simulink model "PID_control_Model_square_input"  (R2022a)
settings: Solver=VariableStepAuto  StartTime=0.0  StopTime=100  RelTol=1e-3
values from neighbouring files (symbols this model uses):
  b1_damp = 0.5    [variable_for_simulink.m]
  b2_damp = 0.5    [variable_for_simulink.m]
  center1 = 0.216    [variable_for_simulink.m]
  center2 = 0.216    [variable_for_simulink.m]
  gravity = 9.8    [variable_for_simulink.m]
  inertia1 = 0.247    [variable_for_simulink.m]
  inertia2 = 0.177    [variable_for_simulink.m]
  length1 = 0.432    [variable_for_simulink.m]
  mass1 = 15.91    [variable_for_simulink.m]
  mass2 = 11.36    [variable_for_simulink.m]
libraries: slpidlib x2
settings Model: Creator=Steve  LastModifiedBy=Steve

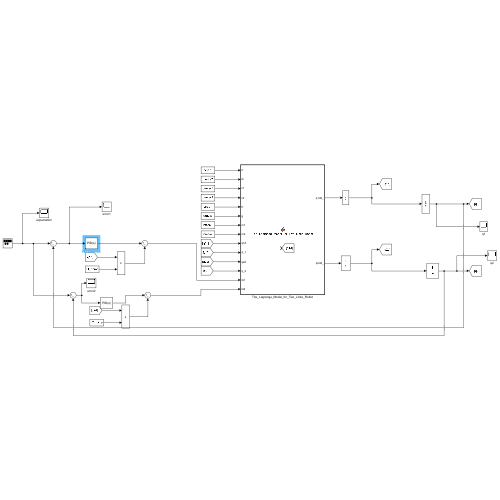
[thumbnail: Simulink's stored preview of the top-level diagram]
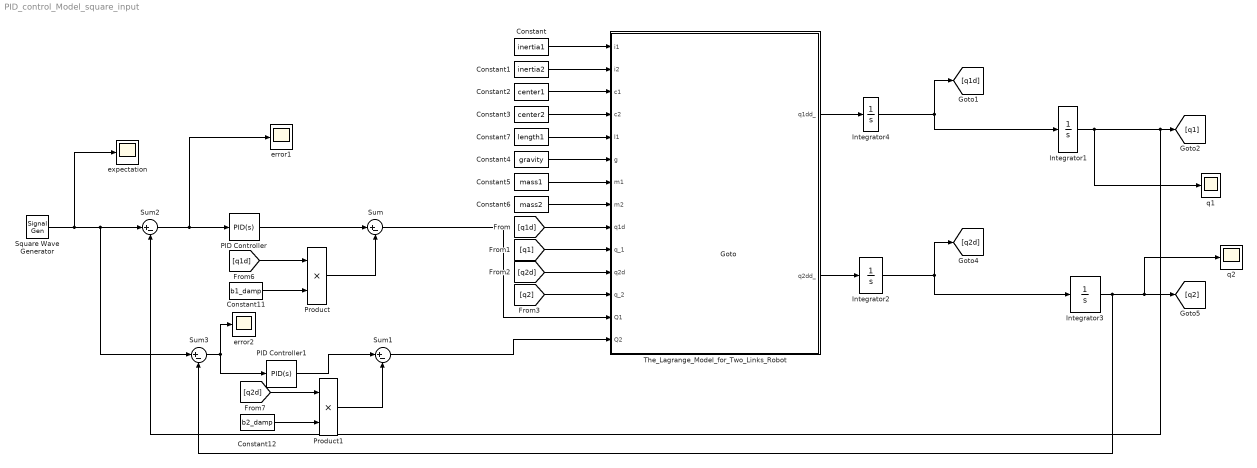
== system PID_control_Model_square_input ==
  Constant : Constant  Value=inertia1
  Constant1 : Constant  Value=inertia2
  Constant11 : Constant  Value=b1_damp
  Constant12 : Constant  Value=b2_damp
  Constant2 : Constant  Value=center1
  Constant3 : Constant  Value=center2
  Constant4 : Constant  Value=gravity
  Constant5 : Constant  Value=mass1
  Constant6 : Constant  Value=mass2
  Constant7 : Constant  Value=length1
  Integrator1 : Integrator  InitialCondition=1
  Integrator2 : Integrator
  Integrator3 : Integrator  InitialCondition=1
  Integrator4 : Integrator
  PID Controller : slpidlib/PID Controller  Controller=PID  Form=Parallel  TimeDomain=Continuous-time  UseExternalTs=off  SampleTime=-1  IntegratorMethod=Forward Euler  FilterMethod=Forward Euler  ControllerParametersSource=internal  P=100  I=50  UseKiTs=off  D=1  N=100  UseFilter=on  TunerSelectOption=Frequency Response Based  InitialConditionSource=internal  InitialConditionForIntegrator=0  InitialConditionForFilter=0  DifferentiatorICPrevScaledInput=0  ExternalReset=none  TrackingMode=off  Kt=1  LimitOutput=off  SatLimitsSource=internal  UpperSaturationLimit=inf  LowerSaturationLimit=-inf  LinearizeAsGain=on  AntiWindupMode=none  Kb=1  POutMin=[]  POutMax=[]  IOutMin=[]  IOutMax=[]  DOutMin=[]  DOutMax=[]  NOutMin=[]  NOutMax=[]  SumOutMin=[]  SumOutMax=[]  SaturationOutMin=[]  SaturationOutMax=[]  PParamMin=[]  PParamMax=[]  IParamMin=[]  IParamMax=[]  DParamMin=[]  DParamMax=[]  NParamMin=[]  NParamMax=[]  KbParamMin=[]  KbParamMax=[]  KtParamMin=[]  KtParamMax=[]  KbOutMin=[]  KbOutMax=[]  KtOutMin=[]  KtOutMax=[]  IntegratorOutMin=[]  IntegratorOutMax=[]  FilterOutMin=[]  FilterOutMax=[]  SumI1OutMin=[]  SumI1OutMax=[]  SumI2OutMin=[]  SumI2OutMax=[]  SumI3OutMin=[]  SumI3OutMax=[]  SumI4OutMin=[]  SumI4OutMax=[]  SumDOutMin=[]  SumDOutMax=[]  DifferentiatorOutMin=[]  DifferentiatorOutMax=[]  FilterDiffOutCoefMin=[]  FilterDiffOutCoefMax=[]  ReciprocalOutMin=[]  ReciprocalOutMax=[]  SumDenOutMin=[]  SumDenOutMax=[]  SumNumOutMin=[]  SumNumOutMax=[]  DivideOutMin=[]  DivideOutMax=[]  UdiffTsProdOutMin=[]  UdiffTsProdOutMax=[]  NTsProdOutMin=[]  NTsProdOutMax=[]  UintegralTsProdOutMin=[]  UintegralTsProdOutMax=[]  UngainTsProdOutMin=[]  UngainTsProdOutMax=[]  IntegratorContinuousStateAttributes=''  IntegratorStateMustResolveToSignalObject=off  IntegratorRTWStateStorageClass=Auto  FilterContinuousStateAttributes=''  FilterStateMustResolveToSignalObject=off  FilterRTWStateStorageClass=Auto  ParallelPVariant=InternalParameters  IdealPVariant=Disabled  IVariant=InternalParameters  DVariant=InternalParameters  IntegratorVariant=Continuous  SatVariant=Disabled  AWVariant=Passthrough  PCopyVariant=Disabled  TRVariant=Disabled  FdbkBlocksVariant=Forward  IdealPFdbkVariant=Disabled  SatFdbkVariant=Disabled  DerivativeFilterVariant=ContFilter  NVariant=InternalParameters  NCopyVariant=Disabled  FilterICVariant=InternalICsFilter  IntegratorICVariant=InternalICs  ExternalResetVariant=Disabled  TRSumVariant=Passthrough  SumFdbkVariant=Disabled  SumVariant=Sum_PID  TsampFilterVariant=InternalTs  TsampNgainVariant=Passthrough  TsampIntegralVariant=Passthrough  ExternalSaturationOutDataTypeStr=Inherit: Same as second input  aMode=0
  PID Controller1 : slpidlib/PID Controller  Controller=PID  Form=Parallel  TimeDomain=Continuous-time  UseExternalTs=off  SampleTime=-1  IntegratorMethod=Forward Euler  FilterMethod=Forward Euler  ControllerParametersSource=internal  P=100  I=50  UseKiTs=off  D=20  N=100  UseFilter=on  TunerSelectOption=Transfer Function Based (PID Tuner App)  InitialConditionSource=internal  InitialConditionForIntegrator=0  InitialConditionForFilter=0  DifferentiatorICPrevScaledInput=0  ExternalReset=none  TrackingMode=off  Kt=1  LimitOutput=off  SatLimitsSource=internal  UpperSaturationLimit=inf  LowerSaturationLimit=-inf  LinearizeAsGain=on  AntiWindupMode=none  Kb=1  POutMin=[]  POutMax=[]  IOutMin=[]  IOutMax=[]  DOutMin=[]  DOutMax=[]  NOutMin=[]  NOutMax=[]  SumOutMin=[]  SumOutMax=[]  SaturationOutMin=[]  SaturationOutMax=[]  PParamMin=[]  PParamMax=[]  IParamMin=[]  IParamMax=[]  DParamMin=[]  DParamMax=[]  NParamMin=[]  NParamMax=[]  KbParamMin=[]  KbParamMax=[]  KtParamMin=[]  KtParamMax=[]  KbOutMin=[]  KbOutMax=[]  KtOutMin=[]  KtOutMax=[]  IntegratorOutMin=[]  IntegratorOutMax=[]  FilterOutMin=[]  FilterOutMax=[]  SumI1OutMin=[]  SumI1OutMax=[]  SumI2OutMin=[]  SumI2OutMax=[]  SumI3OutMin=[]  SumI3OutMax=[]  SumI4OutMin=[]  SumI4OutMax=[]  SumDOutMin=[]  SumDOutMax=[]  DifferentiatorOutMin=[]  DifferentiatorOutMax=[]  FilterDiffOutCoefMin=[]  FilterDiffOutCoefMax=[]  ReciprocalOutMin=[]  ReciprocalOutMax=[]  SumDenOutMin=[]  SumDenOutMax=[]  SumNumOutMin=[]  SumNumOutMax=[]  DivideOutMin=[]  DivideOutMax=[]  UdiffTsProdOutMin=[]  UdiffTsProdOutMax=[]  NTsProdOutMin=[]  NTsProdOutMax=[]  UintegralTsProdOutMin=[]  UintegralTsProdOutMax=[]  UngainTsProdOutMin=[]  UngainTsProdOutMax=[]  IntegratorContinuousStateAttributes=''  IntegratorStateMustResolveToSignalObject=off  IntegratorRTWStateStorageClass=Auto  FilterContinuousStateAttributes=''  FilterStateMustResolveToSignalObject=off  FilterRTWStateStorageClass=Auto  ParallelPVariant=InternalParameters  IdealPVariant=Disabled  IVariant=InternalParameters  DVariant=InternalParameters  IntegratorVariant=Continuous  SatVariant=Disabled  AWVariant=Passthrough  PCopyVariant=Disabled  TRVariant=Disabled  FdbkBlocksVariant=Forward  IdealPFdbkVariant=Disabled  SatFdbkVariant=Disabled  DerivativeFilterVariant=ContFilter  NVariant=InternalParameters  NCopyVariant=Disabled  FilterICVariant=InternalICsFilter  IntegratorICVariant=InternalICs  ExternalResetVariant=Disabled  TRSumVariant=Passthrough  SumFdbkVariant=Disabled  SumVariant=Sum_PID  TsampFilterVariant=InternalTs  TsampNgainVariant=Passthrough  TsampIntegralVariant=Passthrough  ExternalSaturationOutDataTypeStr=Inherit: Same as second input  aMode=0
  Product : Product
  Product1 : Product
  Square Wave Generator : SignalGenerator  WaveForm=square  Units=rad/sec
  Sum{,1..3} (4 alike) : Sum  Inputs=|+-
  The_Lagrange_Model_for_Two_Links_Robot : MATLAB Function  TreatAsAtomicUnit=on
  error1 : Scope
  error2 : Scope
  expectation : Scope
  q1 : Scope
  q2 : Scope
  wires:
  Constant4/1 -> The_Lagrange_Model_for_Two_Links_Robot/6(g)
  Constant1/1 -> The_Lagrange_Model_for_Two_Links_Robot/2(i2)
  Constant3/1 -> The_Lagrange_Model_for_Two_Links_Robot/4(c2)
  Constant/1 -> The_Lagrange_Model_for_Two_Links_Robot/1(i1)
  Constant2/1 -> The_Lagrange_Model_for_Two_Links_Robot/3(c1)
  Constant7/1 -> The_Lagrange_Model_for_Two_Links_Robot/5(l1)
  Constant5/1 -> The_Lagrange_Model_for_Two_Links_Robot/7(m1)
  Constant6/1 -> The_Lagrange_Model_for_Two_Links_Robot/8(m2)
  [q1d] -> The_Lagrange_Model_for_Two_Links_Robot/9(q1d)
  [q1] -> The_Lagrange_Model_for_Two_Links_Robot/10(q_1)
  [q2d] -> The_Lagrange_Model_for_Two_Links_Robot/11(q2d)
  [q2] -> The_Lagrange_Model_for_Two_Links_Robot/12(q_2)
  Integrator4/1 -> [q1d], Integrator1/1
  [q2d] -> Product1/1
  Integrator2/1 -> Integrator3/1, [q2d]
  Constant12/1 -> Product1/2
  Integrator1/1 -> Sum2/2, [q1], q1/1
  Integrator3/1 -> [q2], q2/1, Sum3/2
  Product/1 -> Sum/2
  [q1d] -> Product/1
  Constant11/1 -> Product/2
  Product1/1 -> Sum1/2
  The_Lagrange_Model_for_Two_Links_Robot/1(q1dd_) -> Integrator4/1
  The_Lagrange_Model_for_Two_Links_Robot/2(q2dd_) -> Integrator2/1
  Sum/1 -> The_Lagrange_Model_for_Two_Links_Robot/13(Q1)
  Sum1/1 -> The_Lagrange_Model_for_Two_Links_Robot/14(Q2)
  Square Wave Generator/1 -> expectation/1, Sum3/1, Sum2/1
  Sum2/1 -> error1/1, PID Controller/1
  PID Controller/1 -> Sum/1
  Sum3/1 -> error2/1, PID Controller1/1
  PID Controller1/1 -> Sum1/1

== matlab function PID_control_Model_square_input/The_Lagrange_Model_for_Two_Links_Robot ==
  data: i1 input; q1dd_ output; i2 input; c1 input; c2 input; l1 input; g input; m1 input; m2 input; q1d input; q_1 input; q2d input; q_2 input; Q1 input; Q2 input; q2dd_ output
function [q1dd_,q2dd_] = The_Lagrange_Model_for_Two_Links_Robot(i1,i2,c1,c2,l1,g,m1,m2,q1d,q_1,q2d,q_2,Q1,Q2)
%#codegen

%    This function was generated by the Symbolic Math Toolbox version 9.1.
%    30-Nov-2022 10:42:33

et1 = 1.0./(i1.*i2+i2.*l1.^2.*m2+c2.^2.*l1.^2.*m2.^2+c1.^2.*i2.*m1+c2.^2.*i1.*m2+c1.^2.*c2.^2.*m1.*m2-c2.^2.*l1.^2.*m2.^2.*cos(q_2).^2);
et2 = Q1.*i2-Q2.*i2+Q1.*c2.^2.*m2-Q2.*c2.^2.*m2+c2.^3.*l1.*m2.^2.*q1d.^2.*sin(q_2)+c2.^3.*l1.*m2.^2.*q2d.^2.*sin(q_2)-c2.^2.*g.*l1.*m2.^2.*cos(q_1)-Q2.*c2.*l1.*m2.*cos(q_2)-c1.*g.*i2.*m1.*cos(q_1)-g.*i2.*l1.*m2.*cos(q_1)+c2.^3.*l1.*m2.^2.*q1d.*q2d.*sin(q_2).*2.0+c2.^2.*g.*l1.*m2.^2.*cos(q_1+q_2).*cos(q_2)+c2.^2.*l1.^2.*m2.^2.*q1d.^2.*cos(q_2).*sin(q_2)-c1.*c2.^2.*g.*m1.*m2.*cos(q_1)+c2.*i2.*l1.*m2.*q1d.^2.*sin(q_2)+c2.*i2.*l1.*m2.*q2d.^2.*sin(q_2)+c2.*i2.*l1.*m2.*q1d.*q2d.*sin(q_2).*2.0;
q1dd_ = et1.*et2;
if nargout > 1
    et3 = Q1.*i2-Q2.*i1-Q2.*i2-Q2.*c1.^2.*m1+Q1.*c2.^2.*m2-Q2.*c2.^2.*m2-Q2.*l1.^2.*m2+c2.*l1.^3.*m2.^2.*q1d.^2.*sin(q_2)+c2.^3.*l1.*m2.^2.*q1d.^2.*sin(q_2)+c2.^3.*l1.*m2.^2.*q2d.^2.*sin(q_2)+c2.*g.*l1.^2.*m2.^2.*cos(q_1+q_2)-c2.^2.*g.*l1.*m2.^2.*cos(q_1)+c2.*g.*i1.*m2.*cos(q_1+q_2)+Q1.*c2.*l1.*m2.*cos(q_2)-Q2.*c2.*l1.*m2.*cos(q_2).*2.0-c1.*g.*i2.*m1.*cos(q_1)-g.*i2.*l1.*m2.*cos(q_1)+c2.^3.*l1.*m2.^2.*q1d.*q2d.*sin(q_2).*2.0+c2.^2.*g.*l1.*m2.^2.*cos(q_1+q_2).*cos(q_2)+c2.^2.*l1.^2.*m2.^2.*q1d.^2.*cos(q_2).*sin(q_2).*2.0;
    et4 = c2.^2.*l1.^2.*m2.^2.*q2d.^2.*cos(q_2).*sin(q_2)-c2.*g.*l1.^2.*m2.^2.*cos(q_1).*cos(q_2)+c1.^2.*c2.*g.*m1.*m2.*cos(q_1+q_2)-c1.*c2.^2.*g.*m1.*m2.*cos(q_1)+c2.*i1.*l1.*m2.*q1d.^2.*sin(q_2)+c2.*i2.*l1.*m2.*q1d.^2.*sin(q_2)+c2.*i2.*l1.*m2.*q2d.^2.*sin(q_2)+c2.^2.*l1.^2.*m2.^2.*q1d.*q2d.*cos(q_2).*sin(q_2).*2.0+c1.^2.*c2.*l1.*m1.*m2.*q1d.^2.*sin(q_2)+c2.*i2.*l1.*m2.*q1d.*q2d.*sin(q_2).*2.0-c1.*c2.*g.*l1.*m1.*m2.*cos(q_1).*cos(q_2);
    q2dd_ = -(et3+et4)./(i1.*i2+i2.*l1.^2.*m2+c2.^2.*l1.^2.*m2.^2+c1.^2.*i2.*m1+c2.^2.*i1.*m2+c1.^2.*c2.^2.*m1.*m2-c2.^2.*l1.^2.*m2.^2.*cos(q_2).^2);
end
